simulink model "p2_4"  (R2017b)
settings: Solver=VariableStepAuto  StartTime=0.0  StopTime=500  RelTol=1e-3
values from neighbouring files (symbols this model uses):
  g = 9.8    [CodeControlProject2.m]    (also in linear_system.m = 9.81; main.m; nonlinear_system.m = 9.81)
  K = lqr(A,B,Q,R)    [CodeControlProject2.m]
  l1 = 20    [CodeControlProject2.m]
  l2 = 10    [CodeControlProject2.m]
  M = 1000    [CodeControlProject2.m]    (also in main.m)
  m1 = 100    [CodeControlProject2.m]
  m2 = 100    [CodeControlProject2.m]
settings Model: Creator=srini  LastModifiedBy=srini

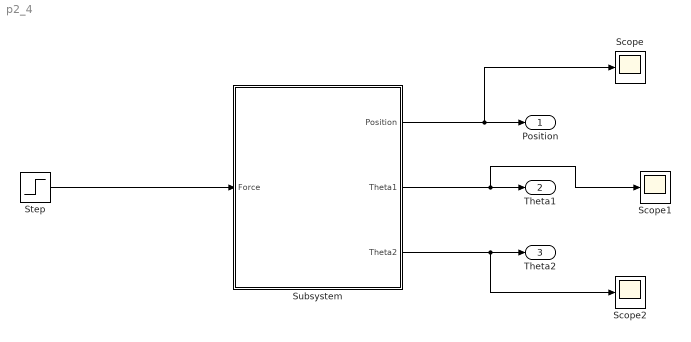
== system p2_4 ==
  Scope : Scope
  Scope1 : Scope
  Scope2 : Scope
  Step : Step  SampleTime=0
  Subsystem : Subsystem
  Position : Outport
  Theta1 : Outport  Port=2
  Theta2 : Outport  Port=3
  wires:
  Subsystem/1(Position) -> Scope/1, Position/1
  Subsystem/2(Theta1) -> Scope1/1, Theta1/1
  Subsystem/3(Theta2) -> Scope2/1, Theta2/1
  Step/1 -> Subsystem/1(Force)

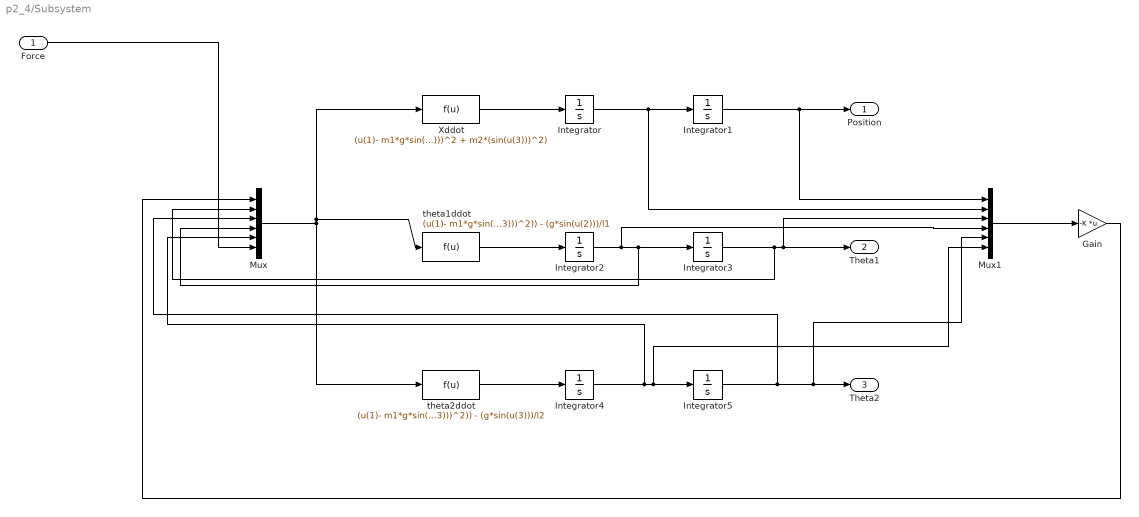
== system p2_4/Subsystem ==
  Force : Inport
  Gain : Gain  Gain=-K  Multiplication=Matrix(K*u)
  Integrator{,1..5} (6 alike) : Integrator
  Mux : Mux  Inputs=6
  Mux1 : Mux  Inputs=6
  Xddot : Fcn  Expr=(u(1)- m1*g*sin(u(2))*cos(u(2)) - m1*l1*sin(u(2))*(u(4))^2 - m2*g*sin(u(3))*cos(u(3)) - m2*l2*sin(u(3))*(u(5))^2)/(M + m1*(sin(u(2)))^2 + m2*(sin(u(3)))^2)
  theta1ddot : Fcn  Expr=(u(1)- m1*g*sin(u(2))*cos(u(2)) - m1*l1*sin(u(2))*(u(4))^2 - m2*g*sin(u(3))*cos(u(3)) - m2*l2*sin(u(3))*(u(5))^2)*cos(u(2))/(l1*(M + m1*(sin(u(2)))^2 + m2*(sin(u(3)))^2)) - (g*sin(u(2)))/l1
  theta2ddot : Fcn  Expr=(u(1)- m1*g*sin(u(2))*cos(u(2)) - m1*l1*sin(u(2))*(u(4))^2 - m2*g*sin(u(3))*cos(u(3)) - m2*l2*sin(u(3))*(u(5))^2)*cos(u(3))/(l2*(M + m1*(sin(u(2)))^2 + m2*(sin(u(3)))^2)) - (g*sin(u(3)))/l2
  Position : Outport
  Theta1 : Outport  Port=2
  Theta2 : Outport  Port=3
  wires:
  Integrator1/1 -> Mux1/1, Position/1
  Integrator/1 -> Mux1/2, Integrator1/1
  Mux/1 -> theta1ddot/1, Xddot/1, theta2ddot/1
  Xddot/1 -> Integrator/1
  theta2ddot/1 -> Integrator4/1
  theta1ddot/1 -> Integrator2/1
  Integrator2/1 -> Mux1/4, Mux/4, Integrator3/1
  Integrator5/1 -> Mux1/5, Theta2/1, Mux/3
  Integrator3/1 -> Mux1/3, Theta1/1, Mux/2
  Integrator4/1 -> Mux/5, Mux1/6, Integrator5/1
  Mux1/1 -> Gain/1
  Gain/1 -> Mux/1
  Force/1 -> Mux/6
